simulink model "red_adelanto_1_ao"  (R2020b)
settings: Solver=VariableStepAuto  StartTime=0.0  StopTime=t(end)  MaxStep=1e-4  RelTol=1e-3
PreLoadFcn:
  | amp_op_tarea_f
InitFcn:
  | amp_op_tarea_f
values from neighbouring files (symbols this model uses):
  C1 = 10e-6    (= 1e-05)    [compensador_adelanto.m]
  C2 = C1    (= 1e-05)    [compensador_adelanto.m]
  R1 = 1/(8*C)    (= 12500)    [compensador_adelanto.m]
  R2 = K/C    [compensador_adelanto.m]
  R3 = 10e3    (= 10000)    [compensador_adelanto.m]
undefined symbols (not defined in the file or in its folder): Rf, Ri
settings Model: Creator=carma  LastModifiedBy=carma

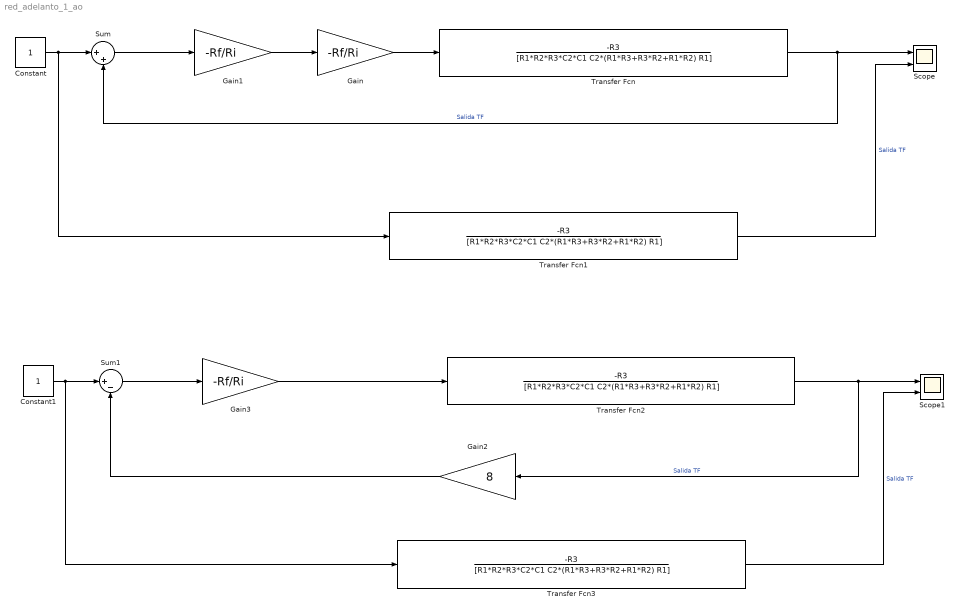
== system red_adelanto_1_ao ==
  Constant : Constant  VectorParams1D=off  SampleTime=-1
  Constant1 : Constant  VectorParams1D=off  SampleTime=-1
  Gain : Gain  Gain=-Rf/Ri
  Gain1 : Gain  Gain=-Rf/Ri
  Gain2 : Gain  Gain=8
  Gain3 : Gain  Gain=-Rf/Ri
  Scope : Scope  NumInputPorts=2
  Scope1 : Scope  NumInputPorts=2
  Sum : Sum  Inputs=|++
  Sum1 : Sum  Inputs=|+-
  Transfer Fcn{,1..3} (4 alike) : TransferFcn  Numerator=-R3  Denominator=[R1*R2*R3*C2*C1 C2*(R1*R3+R3*R2+R1*R2) R1]
  wires:
  Gain/1 -> Transfer Fcn/1
  Transfer Fcn/1 -> Sum/2, Scope/1  "Salida TF"
  Gain1/1 -> Gain/1
  Sum/1 -> Gain1/1
  Constant/1 -> Transfer Fcn1/1, Sum/1
  Transfer Fcn1/1 -> Scope/2  "Salida TF"
  Constant1/1 -> Transfer Fcn3/1, Sum1/1
  Sum1/1 -> Gain3/1
  Gain3/1 -> Transfer Fcn2/1
  Transfer Fcn2/1 -> Gain2/1, Scope1/1  "Salida TF"
  Transfer Fcn3/1 -> Scope1/2  "Salida TF"
  Gain2/1 -> Sum1/2
